simulink model "Counter"  (Simulink 8.5)
settings: Solver=FixedStepDiscrete  StartTime=0.0  StopTime=20.0  FixedStep=1.0  RelTol=1e-3
settings Model: Creator=arnaud  LastModifiedBy=Teme  CovSFcnEnable=off
settings DebuggingCC: SolverPrmCheckMsg=warning  FcnCallInpInsideContextMsg=UseLocalSettings

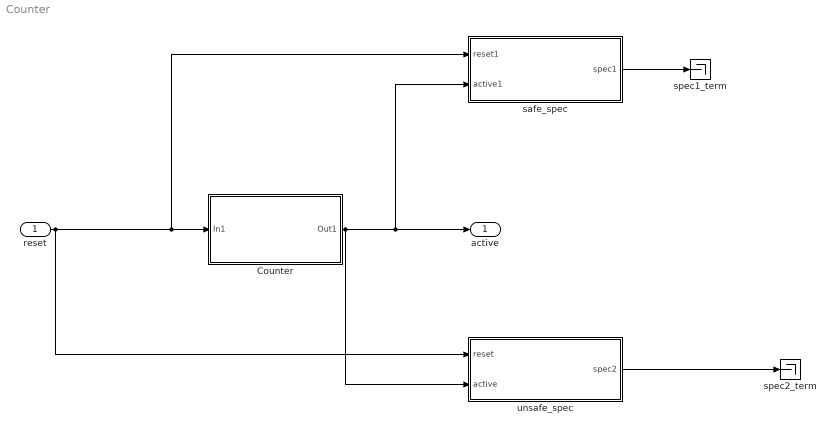
== system Counter ==
  reset : Inport  OutDataTypeStr=boolean
  Counter : Subsystem
  safe_spec : Subsystem  TreatAsAtomicUnit=on  mask(Observer){AnnotationType=ensures, ObserverType=[]}
      mask prompts: AnnotationType "Type of annotation (pre/post...)"; ObserverType "Observer type"
      mask help:
      | Set an observer for the system.
      | The annotation type parameter sets the type of observer:
      | - requires : pre-condition
      | - ensures : post-condition
      | - assert : an assertion
      | - observer : the observer computes a special type of properties
      mask TypeOptions AnnotationType: ensures | requires | assert | observer
      mask Callback AnnotationType:
      | paramStr = get_param(gcb, 'MaskValues');
      | if strcmp(paramStr{1}(1),'o')
      | set_param(gcb,'MaskVisibilities',{'on';'on'});
      | paramStr{2} = 'ellipsoid';
      | set_param(gcb,'MaskValues',paramStr);
      | else
      | set_param(gcb,'MaskVisibilities',{'on';'off'});
      | end
      | clear paramStr;
      mask Callback ObserverType:
      | paramStr = get_param(gcb, 'MaskValues');
      | if strcmp(paramStr{1}(1),'o')
      | set_param(gcb,'MaskVisibilities',{'on';'on'});
      | paramStr{2} = 'ellipsoid';
      | set_param(gcb,'MaskValues',paramStr);
      | else
      | set_param(gcb,'MaskVisibilities',{'on';'off'});
      | end
      | clear paramStr;
      mask Display:
      | color('red')
      | text(0.5, 0.5, ['CoCoSpec: ''' get_param(gcb,'name') ''''], 'horizontalAlignment', 'center');
      | text(0.99, 0.03, '{\bf\fontsize{12}TO BE VERIFIED}', 'hor', 'right', 'ver', 'bottom', 'texmode', 'on');
  spec1_term : Terminator
  spec2_term : Terminator
  unsafe_spec : Subsystem  TreatAsAtomicUnit=on  mask(Observer){AnnotationType=ensures, ObserverType=[]}
      mask prompts: AnnotationType "Type of annotation (pre/post...)"; ObserverType "Observer type"
      mask help:
      | Set an observer for the system.
      | The annotation type parameter sets the type of observer:
      | - requires : pre-condition
      | - ensures : post-condition
      | - assert : an assertion
      | - observer : the observer computes a special type of properties
      mask TypeOptions AnnotationType: ensures | requires | assert | observer
      mask Callback AnnotationType:
      | paramStr = get_param(gcb, 'MaskValues');
      | if strcmp(paramStr{1}(1),'o')
      | set_param(gcb,'MaskVisibilities',{'on';'on'});
      | paramStr{2} = 'ellipsoid';
      | set_param(gcb,'MaskValues',paramStr);
      | else
      | set_param(gcb,'MaskVisibilities',{'on';'off'});
      | end
      | clear paramStr;
      mask Callback ObserverType:
      | paramStr = get_param(gcb, 'MaskValues');
      | if strcmp(paramStr{1}(1),'o')
      | set_param(gcb,'MaskVisibilities',{'on';'on'});
      | paramStr{2} = 'ellipsoid';
      | set_param(gcb,'MaskValues',paramStr);
      | else
      | set_param(gcb,'MaskVisibilities',{'on';'off'});
      | end
      | clear paramStr;
      mask Display:
      | color('red')
      | text(0.5, 0.5, ['CoCoSpec: ''' get_param(gcb,'name') ''''], 'horizontalAlignment', 'center');
      | text(0.99, 0.03, '{\bf\fontsize{12}TO BE VERIFIED}', 'hor', 'right', 'ver', 'bottom', 'texmode', 'on');
  active : Outport
  wires:
  reset/1 -> unsafe_spec/1(reset), safe_spec/1(reset1), Counter/1(In1)
  Counter/1(Out1) -> unsafe_spec/2(active), active/1, safe_spec/2(active1)
  safe_spec/1("spec1  ") -> spec1_term/1
  unsafe_spec/1(spec2) -> spec2_term/1

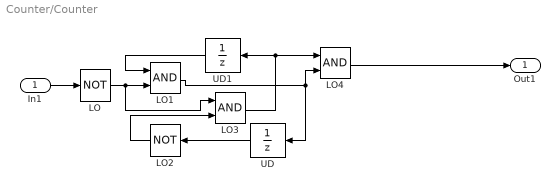
== system Counter/Counter ==
  In1 : Inport
  LO : Logic  Operator=NOT  AllPortsSameDT=off  OutDataTypeStr=boolean
  LO1 : Logic  AllPortsSameDT=off  OutDataTypeStr=boolean
  LO2 : Logic  Operator=NOT  AllPortsSameDT=off  OutDataTypeStr=boolean
  LO3 : Logic  AllPortsSameDT=off  OutDataTypeStr=boolean
  LO4 : Logic  AllPortsSameDT=off  OutDataTypeStr=boolean
  UD : UnitDelay  InitialCondition=false
  UD1 : UnitDelay  InitialCondition=false
  Out1 : Outport
  wires:
  LO4/1 -> Out1/1
  LO/1 -> LO1/2, LO3/1
  LO3/1 -> UD1/1, LO4/1
  In1/1 -> LO/1
  UD/1 -> LO2/1
  LO1/1 -> UD/1, LO4/2
  UD1/1 -> LO1/1
  LO2/1 -> LO3/2

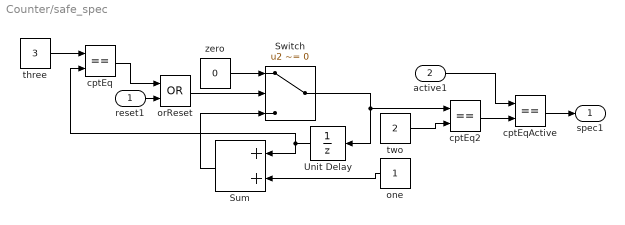
== system Counter/safe_spec ==
  reset1 : Inport
  active1 : Inport  Port=2
  Sum : Sum
  Switch : Switch  Criteria=u2 ~= 0
  Unit Delay : UnitDelay
  cptEq : RelationalOperator  Operator===  OutDataTypeStr=boolean
  cptEq2 : RelationalOperator  Operator===  OutDataTypeStr=boolean
  cptEqActive : RelationalOperator  Operator===  OutDataTypeStr=boolean
  one : Constant
  orReset : Logic  Operator=OR  AllPortsSameDT=off  OutDataTypeStr=boolean
  three : Constant  Value=3
  two : Constant  Value=2
  zero : Constant  Value=0
  "spec1  " : Outport
  wires:
  zero/1 -> Switch/1
  two/1 -> cptEq2/2
  cptEq2/1 -> cptEqActive/2
  active1/1 -> cptEqActive/1
  reset1/1 -> orReset/2
  cptEq/1 -> orReset/1
  orReset/1 -> Switch/2
  Switch/1 -> Unit Delay/1, cptEq2/1
  Unit Delay/1 -> Sum/1, cptEq/2
  one/1 -> Sum/2
  Sum/1 -> Switch/3
  three/1 -> cptEq/1
  cptEqActive/1 -> "spec1  "/1

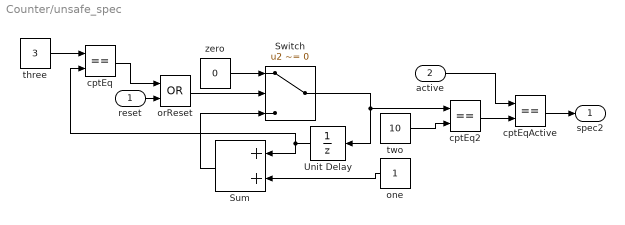
== system Counter/unsafe_spec ==
  reset : Inport
  active : Inport  Port=2
  Sum : Sum
  Switch : Switch  Criteria=u2 ~= 0
  Unit Delay : UnitDelay
  cptEq : RelationalOperator  Operator===  OutDataTypeStr=boolean
  cptEq2 : RelationalOperator  Operator===  OutDataTypeStr=boolean
  cptEqActive : RelationalOperator  Operator===  OutDataTypeStr=boolean
  one : Constant
  orReset : Logic  Operator=OR  AllPortsSameDT=off  OutDataTypeStr=boolean
  three : Constant  Value=3
  two : Constant  Value=10
  zero : Constant  Value=0
  spec2 : Outport
  wires:
  zero/1 -> Switch/1
  two/1 -> cptEq2/2
  cptEq2/1 -> cptEqActive/2
  active/1 -> cptEqActive/1
  reset/1 -> orReset/2
  cptEq/1 -> orReset/1
  orReset/1 -> Switch/2
  Switch/1 -> Unit Delay/1, cptEq2/1
  Unit Delay/1 -> Sum/1, cptEq/2
  one/1 -> Sum/2
  Sum/1 -> Switch/3
  three/1 -> cptEq/1
  cptEqActive/1 -> spec2/1
